simulink model "gm_MATE_HDLsolver_myFirstCircuit"  (R2024b)
settings: Solver=FixedStepDiscrete  StartTime=0.0  StopTime=0.05  FixedStep=6.02409638554217e-09  MaxStep=100e-6  RelTol=1e-4
PostLoadFcn:
  | Ts=1e-6; nb_sw=3; nb_lc=2;nb_r=1;nb_src=1; nb_out=3; rL=1.2;rC=100;L=1e-3; C=1e-5; LpejoSw=1e-6;h=Ts; MAX_INPUTS=16;
  | MAX_OUTPUTS=16;
  | MAX_SWITCHES=8;
  | MAX_INPUTS=16;
InitFcn:
  | Ts=1e-6; nb_sw=3; nb_lc=2;nb_r=1;nb_src=1; nb_out=3; rL=1.2;rC=100;L=1e-3; C=1e-5; LpejoSw=1e-6;h=Ts; MAX_INPUTS=16;
  | MAX_OUTPUTS=16;
  | MAX_SWITCHES=8;
  | MAX_INPUTS=16;
undefined symbols (not defined in the file or in its folder): MATE_SOC
libraries: fl_lib x31, nesl_utility x13, hdlmdlgenlib x10, simetranss x5, simulink x4, hdlsllib x3, ee_lib x2, eeGeneralControl x1
(part 3 of 8)

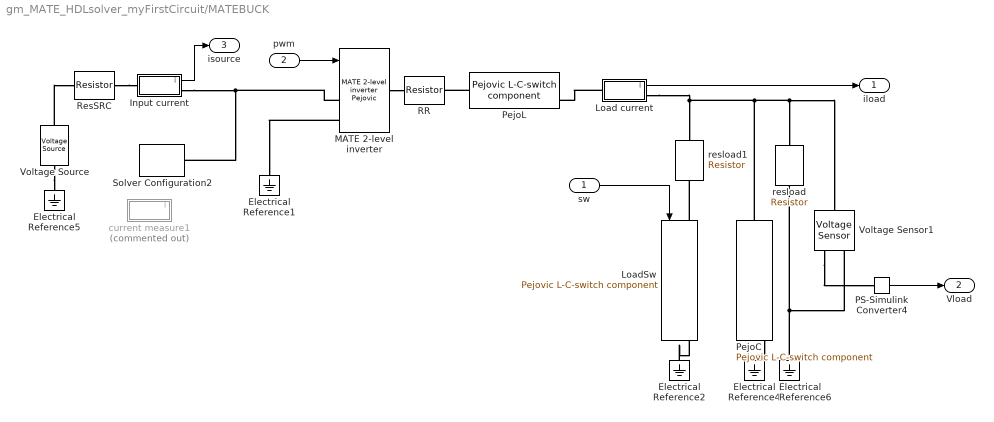
== system gm_MATE_HDLsolver_myFirstCircuit/MATEBUCK ==
  sw : Inport
  pwm : Inport  Port=2
  Electrical Reference{1..2,4..6} (5 alike) : fl_lib/Electrical/Electrical Elements/Electrical Reference
  Input current : Subsystem
  Load current : Subsystem
  LoadSw : simetranss/FPGA/Pejovic L-C-switch component  typ=Switch  Lon=LpejoSw  L=L  C=C  otherSW='coming soon'  Ts=Ts  pcbp=off
  MATE 2-level inverter : simetranss/FPGA/MATE 2-level inverter Pejovic  Lon=1e-6  Ts=Ts
  PS-Simulink Converter4 : nesl_utility/PS-Simulink Converter  PhysicalDomain=network_engine_domain  SubClassName=ps_output  LeftPortType=input  RightPortType=output  PseudoPeriodic=off  Frequencies=[]  VectorFormat=inherit  Unit=inherit  AffineConversion=off
  PejoC : simetranss/FPGA/Pejovic L-C-switch component  typ=Capacitor  Lon=LpejoSw  L=L  C=C  otherSW='coming soon'  Ts=Ts  pcbp=off
  PejoL : simetranss/FPGA/Pejovic L-C-switch component  typ=Inductor  Lon=LpejoSw  L=L  C=C  otherSW='coming soon'  Ts=Ts  pcbp=off
  RR : fl_lib/Electrical/Electrical Elements/Resistor  R=rL Ohm  i_specify=off  i_priority=None  i=0 A  i_nominal_specify=off  i_nominal_value=1  i_nominal_unit=A  v_specify=off  v_priority=None  v=0 V  v_nominal_specify=off  v_nominal_value=1  v_nominal_unit=V
  ResSRC : fl_lib/Electrical/Electrical Elements/Resistor  R=0.01 Ohm  i_specify=off  i_priority=None  i=0 A  i_nominal_specify=off  i_nominal_value=1  i_nominal_unit=A  v_specify=off  v_priority=None  v=0 V  v_nominal_specify=off  v_nominal_value=1  v_nominal_unit=V
  Solver Configuration2 : nesl_utility/Solver Configuration  PhysicalDomain=network_engine_domain  SubClassName=solver  LeftPortType=input  RightPortType=generic  Tones=[]  Harmonics=[]  SimulateNoise=off  Profile=off  UseLocalSampling=off  EnableSwitchedLinearOptims=on  FrequencyDomain=off  UseCCode=off  RelTol=0.001  AbsTol=0.001  MinStep=1e-09  ToWorkspace=off  RevertToSquareIcSolve=off  NumHomotopyIterations=100  PhasorMode=off  PhasorModeNumHarmonics=1  ConsistencySolver=NEWTON_XTOL_AFTER_FTOL  IndexReductionMethod=DerivativeReplacement  DoDC=off  ResidualTolerance=1e-09  ConsistencyTolSource=GLOBAL  ConsistencyAbsTol=0.001  ConsistencyRelTol=0.001  ConsistencyTolFactor=0.001  UseLocalSolver=on  LocalSolverChoice=NE_BACKWARD_EULER_ADVANCER  ResolveIndetEquations=on  FunctionEvalNumThread=1  LocalSolverSampleTime=Ts  DoFixedCost=on  MaxNonlinIter=1  MaxModeIter=2  ComputeImpulses=off  ImpulseIterations=2  LinearAlgebra=auto  LinearAlgebraNumThread=0  EquationFormulation=NE_TIME_EF  DelaysMemoryBudget=1024  AutomaticFiltering=on  FilteringTimeConstant=0.001  PartitionStorageMethod=AS_NEEDED  PartitionMemoryBudget=1024  PartitionMethod=ROBUST  MultibodyUseLocalSolver=off  MultibodyLocalSolverChoice=ODE1  MultibodyLocalSolverSampleTime=0.001
  Voltage Sensor1 : fl_lib/Electrical/Electrical Sensors/Voltage Sensor
  Voltage Source : ee_lib/Sources/Voltage Source  dc_voltage=100 V  ac_voltage=0 V  ac_shift=0 rad  ac_frequency=60 Hz  noise_mode=ee.enum.sources.noise.Disabled  PSD=0 V^2/Hz  sample_time=1e-3 s  repeatability=ee.enum.sources.repeatability.NotRepeatable  user_seed=0  auto_seed=136721035  i_specify=off  i_priority=None  i=0 A  i_nominal_specify=off  i_nominal_value=1  i_nominal_unit=A  v_specify=off  v_priority=None  v=0 V  v_nominal_specify=off  v_nominal_value=1  v_nominal_unit=V
  current measure1 : Subsystem  Commented=on
      mask Display: disp('amp')
  resload : fl_lib/Electrical/Electrical Elements/Resistor  R=rC Ohm  i_specify=off  i_priority=None  i=0 A  i_nominal_specify=off  i_nominal_value=1  i_nominal_unit=A  v_specify=off  v_priority=None  v=0 V  v_nominal_specify=off  v_nominal_value=1  v_nominal_unit=V
  resload1 : fl_lib/Electrical/Electrical Elements/Resistor  R=rC Ohm  i_specify=off  i_priority=None  i=0 A  i_nominal_specify=off  i_nominal_value=1  i_nominal_unit=A  v_specify=off  v_priority=None  v=0 V  v_nominal_specify=off  v_nominal_value=1  v_nominal_unit=V
  iload : Outport
  Vload : Outport  Port=2
  isource : Outport  Port=3
  wires:
  Input current/1(i) -> isource/1
  pwm/1 -> MATE 2-level inverter/1
  Load current/1(i) -> iload/1
  sw/1 -> LoadSw/1
  PS-Simulink Converter4/1 -> Vload/1
  connections:
  ResSRC/RConn1 -- Input current/LConn1
  Electrical Reference2/LConn1 -- LoadSw/RConn1
  LoadSw/LConn1 -- resload1/RConn1
  MATE 2-level inverter/LConn2 -- Electrical Reference1/LConn1
  PejoC/LConn1 -- resload1/LConn1 -- Load current/RConn1 -- resload/LConn1 -- Voltage Sensor1/LConn1
  Solver Configuration2/RConn1 -- MATE 2-level inverter/LConn1 -- Input current/RConn1
  Voltage Sensor1/RConn2 -- resload/RConn1 -- Electrical Reference6/LConn1
  Voltage Sensor1/RConn1 -- PS-Simulink Converter4/LConn1
  PejoC/RConn1 -- Electrical Reference4/LConn1
  PejoL/LConn1 -- RR/RConn1
  MATE 2-level inverter/RConn1 -- RR/LConn1
  Voltage Source/LConn1 -- ResSRC/LConn1
  Voltage Source/RConn1 -- Electrical Reference5/LConn1
  Load current/LConn1 -- PejoL/RConn1

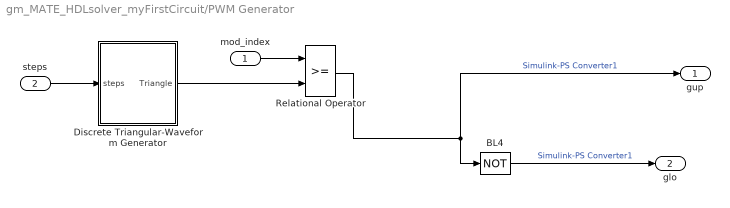
== system gm_MATE_HDLsolver_myFirstCircuit/PWM Generator ==
  mod_index : Inport
  steps : Inport  Port=2
  BL4 : Logic  Operator=NOT  Inputs=1
  Discrete Triangular-Waveform Generator : Subsystem
  Relational Operator : RelationalOperator  OutDataTypeStr=boolean
  gup : Outport  VectorParamsAs1DForOutWhenUnconnected=off
  glo : Outport  Port=2  VectorParamsAs1DForOutWhenUnconnected=off
  wires:
  BL4/1 -> glo/1  "Simulink-PS Converter1"
  Relational Operator/1 -> BL4/1, gup/1  "Simulink-PS Converter1"
  steps/1 -> Discrete Triangular-Waveform Generator/1(steps)
  mod_index/1 -> Relational Operator/1
  Discrete Triangular-Waveform Generator/1(Triangle) -> Relational Operator/2

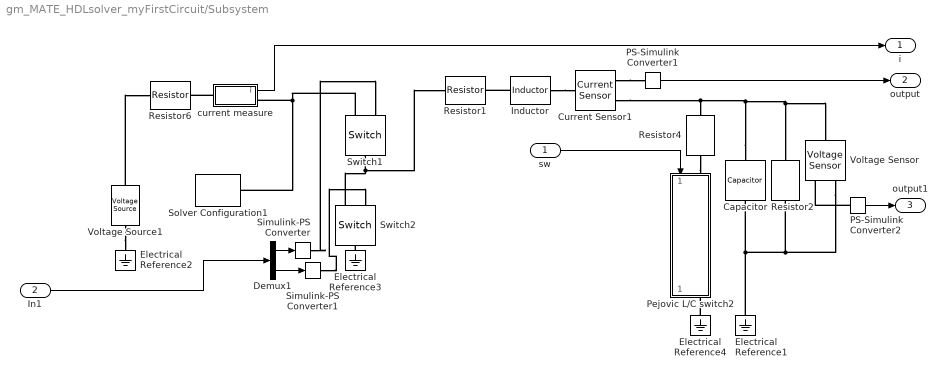
== system gm_MATE_HDLsolver_myFirstCircuit/Subsystem ==
  sw : Inport
  In1 : Inport  Port=2
  Capacitor : fl_lib/Electrical/Electrical Elements/Capacitor  c=C F  r=0 Ohm  g=0 1/Ohm  i_specify=off  i_priority=None  i=0 A  i_nominal_specify=off  i_nominal_value=1  i_nominal_unit=A  v_specify=off  v_priority=None  v=0 V  v_nominal_specify=off  v_nominal_value=1  v_nominal_unit=V  vc_specify=off  vc_priority=High  vc=0 V  vc_nominal_specify=off  vc_nominal_value=1  vc_nominal_unit=V
  Current Sensor1 : fl_lib/Electrical/Electrical Sensors/Current Sensor
  Demux1 : Demux  Outputs=2
  Electrical Reference{1..4} (4 alike) : fl_lib/Electrical/Electrical Elements/Electrical Reference
  Inductor : fl_lib/Electrical/Electrical Elements/Inductor  l=L H  r=0 Ohm  g=1e-9 1/Ohm  i_specify=off  i_priority=None  i=0 A  i_nominal_specify=off  i_nominal_value=1  i_nominal_unit=A  v_specify=off  v_priority=None  v=0 V  v_nominal_specify=off  v_nominal_value=1  v_nominal_unit=V  i_L_specify=off  i_L_priority=High  i_L=0 A  i_L_nominal_specify=off  i_L_nominal_value=1  i_L_nominal_unit=A
  PS-Simulink Converter1 : nesl_utility/PS-Simulink Converter  PhysicalDomain=network_engine_domain  SubClassName=ps_output  LeftPortType=input  RightPortType=output  PseudoPeriodic=off  Frequencies=[]  VectorFormat=inherit  Unit=inherit  AffineConversion=off
  PS-Simulink Converter2 : nesl_utility/PS-Simulink Converter  PhysicalDomain=network_engine_domain  SubClassName=ps_output  LeftPortType=input  RightPortType=output  PseudoPeriodic=off  Frequencies=[]  VectorFormat=inherit  Unit=inherit  AffineConversion=off
  Pejovic L/C switch2 : Subsystem  AncestorBlock=simetranss/FPGA/Pejovic L//C switch  mask(Pejovic Switch){Lon=LpejoSw, Ts=Ts}
      mask prompts: Lon "Selected equivalent ON inductance (H)"; Ts "Sample Time (s)"
      mask help:
      | Pejovic switch model in SimScape
      |
      | Implements a single phase switch model using the Pejovic constant admittance method.
      | The user only has to select the equivalent ON-state inductance of the model, the corresponding Capacitance is computed internally.
      |
      | In the Pejovic model, Ts/Lon=Coff/Ts (Backward Euler) resulting in a constant admittance for the DAE solver.
      |
      | Input signals;
      |
      | gate: the switch gate value (1 for ON , 0 for OFF)
      mask init:
      | Coff=Ts*Ts/Lon;
      | Rsw=Lon/Ts;
      | 
      | if Ts>2e-6
      |     warndlg(['Sample Time of ' num2str(Ts) ' s. may be somehow large for the Pejovic switch to be accurate. Sample time below 2 us are recommended.'])
      | end
      mask Display: disp(['Pswitch'])
  Resistor1 : fl_lib/Electrical/Electrical Elements/Resistor  R=rL Ohm  i_specify=off  i_priority=None  i=0 A  i_nominal_specify=off  i_nominal_value=1  i_nominal_unit=A  v_specify=off  v_priority=None  v=0 V  v_nominal_specify=off  v_nominal_value=1  v_nominal_unit=V
  Resistor2 : fl_lib/Electrical/Electrical Elements/Resistor  R=rC Ohm  i_specify=off  i_priority=None  i=0 A  i_nominal_specify=off  i_nominal_value=1  i_nominal_unit=A  v_specify=off  v_priority=None  v=0 V  v_nominal_specify=off  v_nominal_value=1  v_nominal_unit=V
  Resistor4 : fl_lib/Electrical/Electrical Elements/Resistor  R=rC Ohm  i_specify=off  i_priority=None  i=0 A  i_nominal_specify=off  i_nominal_value=1  i_nominal_unit=A  v_specify=off  v_priority=None  v=0 V  v_nominal_specify=off  v_nominal_value=1  v_nominal_unit=V
  Resistor6 : fl_lib/Electrical/Electrical Elements/Resistor  R=0.01 Ohm  i_specify=off  i_priority=None  i=0 A  i_nominal_specify=off  i_nominal_value=1  i_nominal_unit=A  v_specify=off  v_priority=None  v=0 V  v_nominal_specify=off  v_nominal_value=1  v_nominal_unit=V
  Simulink-PS Converter : nesl_utility/Simulink-PS Converter  PhysicalDomain=network_engine_domain  SubClassName=ps_input  LeftPortType=input  RightPortType=output  PseudoPeriodic=off  Frequencies=[]  NoiseDistribution=none  NoiseParameters=[]  Unit=1  AffineConversion=off  FilteringAndDerivatives=provide  SimscapeFilterOrder=1  InputFilterTimeConstant=0.001  UdotUserProvided=0
  Simulink-PS Converter1 : nesl_utility/Simulink-PS Converter  PhysicalDomain=network_engine_domain  SubClassName=ps_input  LeftPortType=input  RightPortType=output  PseudoPeriodic=off  Frequencies=[]  NoiseDistribution=none  NoiseParameters=[]  Unit=1  AffineConversion=off  FilteringAndDerivatives=provide  SimscapeFilterOrder=1  InputFilterTimeConstant=0.001  UdotUserProvided=0
  Solver Configuration1 : nesl_utility/Solver Configuration  PhysicalDomain=network_engine_domain  SubClassName=solver  LeftPortType=input  RightPortType=generic  Tones=[]  Harmonics=[]  SimulateNoise=off  Profile=off  UseLocalSampling=off  EnableSwitchedLinearOptims=on  FrequencyDomain=off  UseCCode=off  RelTol=0.001  AbsTol=0.001  MinStep=1e-09  ToWorkspace=off  RevertToSquareIcSolve=off  NumHomotopyIterations=100  PhasorMode=off  PhasorModeNumHarmonics=1  ConsistencySolver=NEWTON_XTOL_AFTER_FTOL  IndexReductionMethod=DerivativeReplacement  DoDC=off  ResidualTolerance=1e-09  ConsistencyTolSource=GLOBAL  ConsistencyAbsTol=0.001  ConsistencyRelTol=0.001  ConsistencyTolFactor=0.001  UseLocalSolver=on  LocalSolverChoice=NE_BACKWARD_EULER_ADVANCER  ResolveIndetEquations=on  FunctionEvalNumThread=1  LocalSolverSampleTime=Ts  DoFixedCost=on  MaxNonlinIter=1  MaxModeIter=2  ComputeImpulses=off  ImpulseIterations=2  LinearAlgebra=auto  LinearAlgebraNumThread=0  EquationFormulation=NE_TIME_EF  DelaysMemoryBudget=1024  AutomaticFiltering=on  FilteringTimeConstant=0.001  PartitionStorageMethod=AS_NEEDED  PartitionMemoryBudget=1024  PartitionMethod=ROBUST  MultibodyUseLocalSolver=off  MultibodyLocalSolverChoice=ODE1  MultibodyLocalSolverSampleTime=0.001
  Switch1 : fl_lib/Electrical/Electrical Elements/Switch  R_closed=0.001 Ohm  G_open=1e-8 1/Ohm  Threshold=0.5  i_specify=off  i_priority=None  i=0 A  i_nominal_specify=off  i_nominal_value=1  i_nominal_unit=A  v_specify=off  v_priority=None  v=0 V  v_nominal_specify=off  v_nominal_value=1  v_nominal_unit=V
  Switch2 : fl_lib/Electrical/Electrical Elements/Switch  R_closed=0.001 Ohm  G_open=1e-8 1/Ohm  Threshold=0.5  i_specify=off  i_priority=None  i=0 A  i_nominal_specify=off  i_nominal_value=1  i_nominal_unit=A  v_specify=off  v_priority=None  v=0 V  v_nominal_specify=off  v_nominal_value=1  v_nominal_unit=V
  Voltage Sensor : fl_lib/Electrical/Electrical Sensors/Voltage Sensor
  Voltage Source1 : ee_lib/Sources/Voltage Source  dc_voltage=100 V  ac_voltage=0 V  ac_shift=0 rad  ac_frequency=60 Hz  noise_mode=ee.enum.sources.noise.Disabled  PSD=0 V^2/Hz  sample_time=1e-3 s  repeatability=ee.enum.sources.repeatability.NotRepeatable  user_seed=0  auto_seed=1189375164  i_specify=off  i_priority=None  i=0 A  i_nominal_specify=off  i_nominal_value=1  i_nominal_unit=A  v_specify=off  v_priority=None  v=0 V  v_nominal_specify=off  v_nominal_value=1  v_nominal_unit=V
  current measure : Subsystem
      mask Display: disp('amp')
  i : Outport
  output : Outport  Port=2
  output1 : Outport  Port=3
  wires:
  PS-Simulink Converter2/1 -> output1/1
  PS-Simulink Converter1/1 -> output/1
  In1/1 -> Demux1/1
  Demux1/1 -> Simulink-PS Converter/1
  current measure/1(i) -> i/1
  Demux1/2 -> Simulink-PS Converter1/1
  sw/1 -> Pejovic L/C switch2/1(gate)
  connections:
  Voltage Source1/RConn1 -- Electrical Reference2/LConn1
  Electrical Reference3/LConn1 -- Switch2/LConn1
  Current Sensor1/RConn1 -- PS-Simulink Converter1/LConn1
  Inductor/LConn1 -- Resistor1/RConn1
  Inductor/RConn1 -- Current Sensor1/LConn1
  Simulink-PS Converter1/RConn1 -- Switch2/RConn1
  PS-Simulink Converter2/LConn1 -- Voltage Sensor/RConn1
  Voltage Source1/LConn1 -- Resistor6/LConn1
  current measure/LConn1 -- Resistor6/RConn1
  Resistor4/RConn1 -- Pejovic L/C switch2/LConn1
  Electrical Reference1/LConn1 -- Capacitor/RConn1 -- Resistor2/RConn1 -- Voltage Sensor/RConn2
  Capacitor/LConn1 -- Resistor2/LConn1 -- Voltage Sensor/LConn1 -- Resistor4/LConn1 -- Current Sensor1/RConn2
  Switch1/LConn1 -- Resistor1/LConn1 -- Switch2/RConn2
  Solver Configuration1/RConn1 -- current measure/RConn1 -- Switch1/RConn2
  Simulink-PS Converter/RConn1 -- Switch1/RConn1
  Electrical Reference4/LConn1 -- Pejovic L/C switch2/RConn1

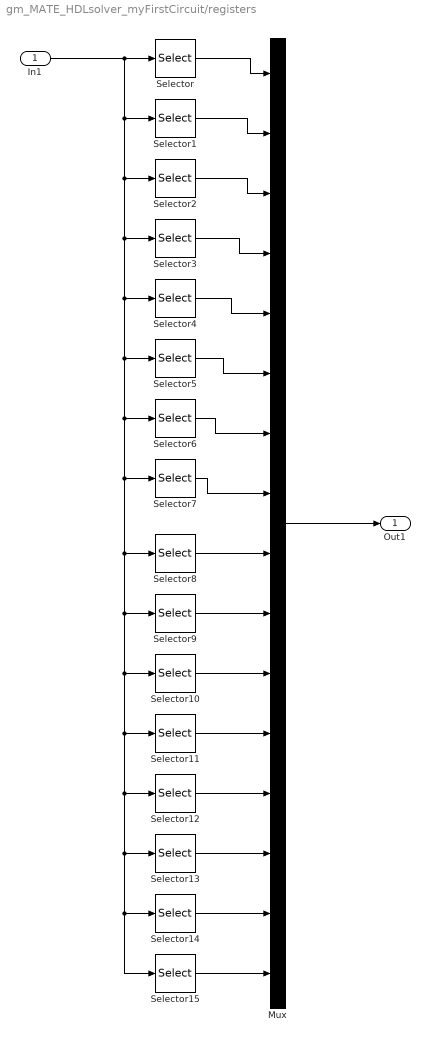
== system gm_MATE_HDLsolver_myFirstCircuit/registers ==
  In1 : Inport
  Mux : Mux  Inputs=16
  Selector : Selector  InputPortWidth=16  IndexOptions=Index vector (dialog)  Indices=1  OutputSizes=1
  Selector1 : Selector  InputPortWidth=16  IndexOptions=Index vector (dialog)  Indices=2  OutputSizes=1
  Selector10 : Selector  InputPortWidth=16  IndexOptions=Index vector (dialog)  Indices=11  OutputSizes=1
  Selector11 : Selector  InputPortWidth=16  IndexOptions=Index vector (dialog)  Indices=12  OutputSizes=1
  Selector12 : Selector  InputPortWidth=16  IndexOptions=Index vector (dialog)  Indices=13  OutputSizes=1
  Selector13 : Selector  InputPortWidth=16  IndexOptions=Index vector (dialog)  Indices=14  OutputSizes=1
  Selector14 : Selector  InputPortWidth=16  IndexOptions=Index vector (dialog)  Indices=15  OutputSizes=1
  Selector15 : Selector  InputPortWidth=16  IndexOptions=Index vector (dialog)  Indices=16  OutputSizes=1
  Selector2 : Selector  InputPortWidth=16  IndexOptions=Index vector (dialog)  Indices=3  OutputSizes=1
  Selector3 : Selector  InputPortWidth=16  IndexOptions=Index vector (dialog)  Indices=4  OutputSizes=1
  Selector4 : Selector  InputPortWidth=16  IndexOptions=Index vector (dialog)  Indices=5  OutputSizes=1
  Selector5 : Selector  InputPortWidth=16  IndexOptions=Index vector (dialog)  Indices=6  OutputSizes=1
  Selector6 : Selector  InputPortWidth=16  IndexOptions=Index vector (dialog)  Indices=7  OutputSizes=1
  Selector7 : Selector  InputPortWidth=16  IndexOptions=Index vector (dialog)  Indices=8  OutputSizes=1
  Selector8 : Selector  InputPortWidth=16  IndexOptions=Index vector (dialog)  Indices=9  OutputSizes=1
  Selector9 : Selector  InputPortWidth=16  IndexOptions=Index vector (dialog)  Indices=10  OutputSizes=1
  Out1 : Outport
  wires:
  Mux/1 -> Out1/1
  Selector7/1 -> Mux/8
  Selector6/1 -> Mux/7
  Selector5/1 -> Mux/6
  Selector4/1 -> Mux/5
  Selector3/1 -> Mux/4
  Selector2/1 -> Mux/3
  Selector1/1 -> Mux/2
  Selector/1 -> Mux/1
  Selector15/1 -> Mux/16
  Selector14/1 -> Mux/15
  Selector13/1 -> Mux/14
  Selector12/1 -> Mux/13
  Selector11/1 -> Mux/12
  Selector10/1 -> Mux/11
  Selector9/1 -> Mux/10
  Selector8/1 -> Mux/9
  In1/1 -> Selector14/1, Selector15/1, Selector13/1, Selector12/1, Selector11/1, Selector10/1, Selector9/1, Selector8/1, Selector7/1, Selector6/1, Selector5/1, Selector4/1, Selector3/1, Selector2/1, Selector1/1, Selector/1

== system gm_MATE_HDLsolver_myFirstCircuit/ForFPGA/Compare To Constant ==
  u : Inport  OutDataTypeStr=fixdt(0,8,0,'DataTypeOverride', 'Off')  SampleTime=1e-06
  Compare : RelationalOperator  Operator===  OutDataTypeStr=boolean
  Constant : Constant  DisableCoverage=on  Value=const  OutDataTypeStr=uint8  SampleTime=-1
  y : Outport  SampleTime=1e-06
  wires:
  u/1 -> Compare/1
  Compare/1 -> y/1
  Constant/1 -> Compare/2

== system gm_MATE_HDLsolver_myFirstCircuit/ForFPGA/Counter Free-Running ==
  Force to be scalar : SignalSpecification  OutDataTypeStr=fixdt(0, 4, 0)  Dimensions=1
  Increment Real World : Subsystem  mask(Real World Value Increment){}
      mask help: Simulink:masks:RealWorldValueIncrement_MD
      mask Display: disp('V++')
  Output : Delay  DelayLength=double(1)  InitialCondition=0  SampleTime=1e-06
  Wrap To Zero : Subsystem  mask(Wrap To Zero){Threshold=double(15)}
      mask prompts: Threshold "Simulink:masks:Threshold_MP"
      mask help: Simulink:masks:WrapToZero_MD
  y : Outport  SampleTime=1e-06
  wires:
  Wrap To Zero/1(Y) -> Output/1
  Output/1 -> y/1, Force to be scalar/1
  Increment Real World/1(y) -> Wrap To Zero/1(U)
  Force to be scalar/1 -> Increment Real World/1(u)

== system gm_MATE_HDLsolver_myFirstCircuit/ForFPGA/Dot Product ==
  In1 : Inport
  In2 : Inport  Port=2
  Dot Product : Sum  OutDataTypeStr=single  SampleTime=6.02409638554217e-09
  Dot Product_pd1 : Delay  DelayLength=6
  Out1 : Outport
  wires:
  In1/1 -> Dot Product/1
  In2/1 -> Dot Product/2
  Dot Product/1 -> Dot Product_pd1/1
  Dot Product_pd1/1 -> Out1/1

== system gm_MATE_HDLsolver_myFirstCircuit/ForFPGA/Dot Product1 ==
  In1 : Inport
  In2 : Inport  Port=2
  Dot Product1 : Sum  OutDataTypeStr=single  SampleTime=6.02409638554217e-09
  Dot Product1_pd1 : Delay  DelayLength=6
  Out1 : Outport
  wires:
  In1/1 -> Dot Product1/1
  In2/1 -> Dot Product1/2
  Dot Product1/1 -> Dot Product1_pd1/1
  Dot Product1_pd1/1 -> Out1/1

== system gm_MATE_HDLsolver_myFirstCircuit/ForFPGA/Dot Product10 ==
  In1 : Inport
  In2 : Inport  Port=2
  Dot Product10 : Sum  OutDataTypeStr=single  SampleTime=6.02409638554217e-09
  Dot Product10_pd1 : Delay  DelayLength=6
  Out1 : Outport
  wires:
  In1/1 -> Dot Product10/1
  In2/1 -> Dot Product10/2
  Dot Product10/1 -> Dot Product10_pd1/1
  Dot Product10_pd1/1 -> Out1/1

== system gm_MATE_HDLsolver_myFirstCircuit/ForFPGA/Dot Product101 ==
  In1 : Inport
  In2 : Inport  Port=2
  Dot Product101 : Sum  OutDataTypeStr=single  SampleTime=6.02409638554217e-09
  Dot Product101_pd1 : Delay  DelayLength=6
  Out1 : Outport
  wires:
  In1/1 -> Dot Product101/1
  In2/1 -> Dot Product101/2
  Dot Product101/1 -> Dot Product101_pd1/1
  Dot Product101_pd1/1 -> Out1/1

== system gm_MATE_HDLsolver_myFirstCircuit/ForFPGA/Dot Product1010 ==
  In1 : Inport
  In2 : Inport  Port=2
  Dot Product1010 : Sum  OutDataTypeStr=single  SampleTime=6.02409638554217e-09
  Dot Product1010_pd1 : Delay  DelayLength=6
  Out1 : Outport
  wires:
  In1/1 -> Dot Product1010/1
  In2/1 -> Dot Product1010/2
  Dot Product1010/1 -> Dot Product1010_pd1/1
  Dot Product1010_pd1/1 -> Out1/1

== system gm_MATE_HDLsolver_myFirstCircuit/ForFPGA/Dot Product1011 ==
  In1 : Inport
  In2 : Inport  Port=2
  Dot Product1011 : Sum  OutDataTypeStr=single  SampleTime=6.02409638554217e-09
  Dot Product1011_pd1 : Delay  DelayLength=6
  Out1 : Outport
  wires:
  In1/1 -> Dot Product1011/1
  In2/1 -> Dot Product1011/2
  Dot Product1011/1 -> Dot Product1011_pd1/1
  Dot Product1011_pd1/1 -> Out1/1

== system gm_MATE_HDLsolver_myFirstCircuit/ForFPGA/Dot Product1012 ==
  In1 : Inport
  In2 : Inport  Port=2
  Dot Product1012 : Sum  OutDataTypeStr=single  SampleTime=6.02409638554217e-09
  Dot Product1012_pd1 : Delay  DelayLength=6
  Out1 : Outport
  wires:
  In1/1 -> Dot Product1012/1
  In2/1 -> Dot Product1012/2
  Dot Product1012/1 -> Dot Product1012_pd1/1
  Dot Product1012_pd1/1 -> Out1/1

== system gm_MATE_HDLsolver_myFirstCircuit/ForFPGA/Dot Product1013 ==
  In1 : Inport
  In2 : Inport  Port=2
  Dot Product1013 : Sum  OutDataTypeStr=single  SampleTime=6.02409638554217e-09
  Dot Product1013_pd1 : Delay  DelayLength=6
  Out1 : Outport
  wires:
  In1/1 -> Dot Product1013/1
  In2/1 -> Dot Product1013/2
  Dot Product1013/1 -> Dot Product1013_pd1/1
  Dot Product1013_pd1/1 -> Out1/1

== system gm_MATE_HDLsolver_myFirstCircuit/ForFPGA/Dot Product1014 ==
  In1 : Inport
  In2 : Inport  Port=2
  Dot Product1014 : Sum  OutDataTypeStr=single  SampleTime=6.02409638554217e-09
  Dot Product1014_pd1 : Delay  DelayLength=6
  Out1 : Outport
  wires:
  In1/1 -> Dot Product1014/1
  In2/1 -> Dot Product1014/2
  Dot Product1014/1 -> Dot Product1014_pd1/1
  Dot Product1014_pd1/1 -> Out1/1

== system gm_MATE_HDLsolver_myFirstCircuit/ForFPGA/Dot Product1015 ==
  In1 : Inport
  In2 : Inport  Port=2
  Dot Product1015 : Sum  OutDataTypeStr=single  SampleTime=6.02409638554217e-09
  Dot Product1015_pd1 : Delay  DelayLength=6
  Out1 : Outport
  wires:
  In1/1 -> Dot Product1015/1
  In2/1 -> Dot Product1015/2
  Dot Product1015/1 -> Dot Product1015_pd1/1
  Dot Product1015_pd1/1 -> Out1/1

== system gm_MATE_HDLsolver_myFirstCircuit/ForFPGA/Dot Product102 ==
  In1 : Inport
  In2 : Inport  Port=2
  Dot Product102 : Sum  OutDataTypeStr=single  SampleTime=6.02409638554217e-09
  Dot Product102_pd1 : Delay  DelayLength=6
  Out1 : Outport
  wires:
  In1/1 -> Dot Product102/1
  In2/1 -> Dot Product102/2
  Dot Product102/1 -> Dot Product102_pd1/1
  Dot Product102_pd1/1 -> Out1/1

== system gm_MATE_HDLsolver_myFirstCircuit/ForFPGA/Dot Product103 ==
  In1 : Inport
  In2 : Inport  Port=2
  Dot Product103 : Sum  OutDataTypeStr=single  SampleTime=6.02409638554217e-09
  Dot Product103_pd1 : Delay  DelayLength=6
  Out1 : Outport
  wires:
  In1/1 -> Dot Product103/1
  In2/1 -> Dot Product103/2
  Dot Product103/1 -> Dot Product103_pd1/1
  Dot Product103_pd1/1 -> Out1/1

== system gm_MATE_HDLsolver_myFirstCircuit/ForFPGA/Dot Product104 ==
  In1 : Inport
  In2 : Inport  Port=2
  Dot Product104 : Sum  OutDataTypeStr=single  SampleTime=6.02409638554217e-09
  Dot Product104_pd1 : Delay  DelayLength=6
  Out1 : Outport
  wires:
  In1/1 -> Dot Product104/1
  In2/1 -> Dot Product104/2
  Dot Product104/1 -> Dot Product104_pd1/1
  Dot Product104_pd1/1 -> Out1/1

== system gm_MATE_HDLsolver_myFirstCircuit/ForFPGA/Dot Product105 ==
  In1 : Inport
  In2 : Inport  Port=2
  Dot Product105 : Sum  OutDataTypeStr=single  SampleTime=6.02409638554217e-09
  Dot Product105_pd1 : Delay  DelayLength=6
  Out1 : Outport
  wires:
  In1/1 -> Dot Product105/1
  In2/1 -> Dot Product105/2
  Dot Product105/1 -> Dot Product105_pd1/1
  Dot Product105_pd1/1 -> Out1/1

== system gm_MATE_HDLsolver_myFirstCircuit/ForFPGA/Dot Product106 ==
  In1 : Inport
  In2 : Inport  Port=2
  Dot Product106 : Sum  OutDataTypeStr=single  SampleTime=6.02409638554217e-09
  Dot Product106_pd1 : Delay  DelayLength=6
  Out1 : Outport
  wires:
  In1/1 -> Dot Product106/1
  In2/1 -> Dot Product106/2
  Dot Product106/1 -> Dot Product106_pd1/1
  Dot Product106_pd1/1 -> Out1/1

== system gm_MATE_HDLsolver_myFirstCircuit/ForFPGA/Dot Product107 ==
  In1 : Inport
  In2 : Inport  Port=2
  Dot Product107 : Sum  OutDataTypeStr=single  SampleTime=6.02409638554217e-09
  Dot Product107_pd1 : Delay  DelayLength=6
  Out1 : Outport
  wires:
  In1/1 -> Dot Product107/1
  In2/1 -> Dot Product107/2
  Dot Product107/1 -> Dot Product107_pd1/1
  Dot Product107_pd1/1 -> Out1/1

== system gm_MATE_HDLsolver_myFirstCircuit/ForFPGA/Dot Product108 ==
  In1 : Inport
  In2 : Inport  Port=2
  Dot Product108 : Sum  OutDataTypeStr=single  SampleTime=6.02409638554217e-09
  Dot Product108_pd1 : Delay  DelayLength=6
  Out1 : Outport
  wires:
  In1/1 -> Dot Product108/1
  In2/1 -> Dot Product108/2
  Dot Product108/1 -> Dot Product108_pd1/1
  Dot Product108_pd1/1 -> Out1/1

== system gm_MATE_HDLsolver_myFirstCircuit/ForFPGA/Dot Product109 ==
  In1 : Inport
  In2 : Inport  Port=2
  Dot Product109 : Sum  OutDataTypeStr=single  SampleTime=6.02409638554217e-09
  Dot Product109_pd1 : Delay  DelayLength=6
  Out1 : Outport
  wires:
  In1/1 -> Dot Product109/1
  In2/1 -> Dot Product109/2
  Dot Product109/1 -> Dot Product109_pd1/1
  Dot Product109_pd1/1 -> Out1/1

== system gm_MATE_HDLsolver_myFirstCircuit/ForFPGA/Dot Product11 ==
  In1 : Inport
  In2 : Inport  Port=2
  Dot Product11 : Sum  OutDataTypeStr=single  SampleTime=6.02409638554217e-09
  Dot Product11_pd1 : Delay  DelayLength=6
  Out1 : Outport
  wires:
  In1/1 -> Dot Product11/1
  In2/1 -> Dot Product11/2
  Dot Product11/1 -> Dot Product11_pd1/1
  Dot Product11_pd1/1 -> Out1/1

== system gm_MATE_HDLsolver_myFirstCircuit/ForFPGA/Dot Product110 ==
  In1 : Inport
  In2 : Inport  Port=2
  Dot Product110 : Sum  OutDataTypeStr=single  SampleTime=6.02409638554217e-09
  Dot Product110_pd1 : Delay  DelayLength=6
  Out1 : Outport
  wires:
  In1/1 -> Dot Product110/1
  In2/1 -> Dot Product110/2
  Dot Product110/1 -> Dot Product110_pd1/1
  Dot Product110_pd1/1 -> Out1/1

== system gm_MATE_HDLsolver_myFirstCircuit/ForFPGA/Dot Product111 ==
  In1 : Inport
  In2 : Inport  Port=2
  Dot Product111 : Sum  OutDataTypeStr=single  SampleTime=6.02409638554217e-09
  Dot Product111_pd1 : Delay  DelayLength=6
  Out1 : Outport
  wires:
  In1/1 -> Dot Product111/1
  In2/1 -> Dot Product111/2
  Dot Product111/1 -> Dot Product111_pd1/1
  Dot Product111_pd1/1 -> Out1/1

== system gm_MATE_HDLsolver_myFirstCircuit/ForFPGA/Dot Product1110 ==
  In1 : Inport
  In2 : Inport  Port=2
  Dot Product1110 : Sum  OutDataTypeStr=single  SampleTime=6.02409638554217e-09
  Dot Product1110_pd1 : Delay  DelayLength=6
  Out1 : Outport
  wires:
  In1/1 -> Dot Product1110/1
  In2/1 -> Dot Product1110/2
  Dot Product1110/1 -> Dot Product1110_pd1/1
  Dot Product1110_pd1/1 -> Out1/1

== system gm_MATE_HDLsolver_myFirstCircuit/ForFPGA/Dot Product1111 ==
  In1 : Inport
  In2 : Inport  Port=2
  Dot Product1111 : Sum  OutDataTypeStr=single  SampleTime=6.02409638554217e-09
  Dot Product1111_pd1 : Delay  DelayLength=6
  Out1 : Outport
  wires:
  In1/1 -> Dot Product1111/1
  In2/1 -> Dot Product1111/2
  Dot Product1111/1 -> Dot Product1111_pd1/1
  Dot Product1111_pd1/1 -> Out1/1

== system gm_MATE_HDLsolver_myFirstCircuit/ForFPGA/Dot Product1112 ==
  In1 : Inport
  In2 : Inport  Port=2
  Dot Product1112 : Sum  OutDataTypeStr=single  SampleTime=6.02409638554217e-09
  Dot Product1112_pd1 : Delay  DelayLength=6
  Out1 : Outport
  wires:
  In1/1 -> Dot Product1112/1
  In2/1 -> Dot Product1112/2
  Dot Product1112/1 -> Dot Product1112_pd1/1
  Dot Product1112_pd1/1 -> Out1/1

== system gm_MATE_HDLsolver_myFirstCircuit/ForFPGA/Dot Product1113 ==
  In1 : Inport
  In2 : Inport  Port=2
  Dot Product1113 : Sum  OutDataTypeStr=single  SampleTime=6.02409638554217e-09
  Dot Product1113_pd1 : Delay  DelayLength=6
  Out1 : Outport
  wires:
  In1/1 -> Dot Product1113/1
  In2/1 -> Dot Product1113/2
  Dot Product1113/1 -> Dot Product1113_pd1/1
  Dot Product1113_pd1/1 -> Out1/1

== system gm_MATE_HDLsolver_myFirstCircuit/ForFPGA/Dot Product1114 ==
  In1 : Inport
  In2 : Inport  Port=2
  Dot Product1114 : Sum  OutDataTypeStr=single  SampleTime=6.02409638554217e-09
  Dot Product1114_pd1 : Delay  DelayLength=6
  Out1 : Outport
  wires:
  In1/1 -> Dot Product1114/1
  In2/1 -> Dot Product1114/2
  Dot Product1114/1 -> Dot Product1114_pd1/1
  Dot Product1114_pd1/1 -> Out1/1

== system gm_MATE_HDLsolver_myFirstCircuit/ForFPGA/Dot Product1115 ==
  In1 : Inport
  In2 : Inport  Port=2
  Dot Product1115 : Sum  OutDataTypeStr=single  SampleTime=6.02409638554217e-09
  Dot Product1115_pd1 : Delay  DelayLength=6
  Out1 : Outport
  wires:
  In1/1 -> Dot Product1115/1
  In2/1 -> Dot Product1115/2
  Dot Product1115/1 -> Dot Product1115_pd1/1
  Dot Product1115_pd1/1 -> Out1/1

== system gm_MATE_HDLsolver_myFirstCircuit/ForFPGA/Dot Product1116 ==
  In1 : Inport
  In2 : Inport  Port=2
  Dot Product1116 : Sum  OutDataTypeStr=single  SampleTime=6.02409638554217e-09
  Dot Product1116_pd1 : Delay  DelayLength=6
  Out1 : Outport
  wires:
  In1/1 -> Dot Product1116/1
  In2/1 -> Dot Product1116/2
  Dot Product1116/1 -> Dot Product1116_pd1/1
  Dot Product1116_pd1/1 -> Out1/1

== system gm_MATE_HDLsolver_myFirstCircuit/ForFPGA/Dot Product1117 ==
  In1 : Inport
  In2 : Inport  Port=2
  Dot Product1117 : Sum  OutDataTypeStr=single  SampleTime=6.02409638554217e-09
  Dot Product1117_pd1 : Delay  DelayLength=6
  Out1 : Outport
  wires:
  In1/1 -> Dot Product1117/1
  In2/1 -> Dot Product1117/2
  Dot Product1117/1 -> Dot Product1117_pd1/1
  Dot Product1117_pd1/1 -> Out1/1

== system gm_MATE_HDLsolver_myFirstCircuit/ForFPGA/Dot Product1118 ==
  In1 : Inport
  In2 : Inport  Port=2
  Dot Product1118 : Sum  OutDataTypeStr=single  SampleTime=6.02409638554217e-09
  Dot Product1118_pd1 : Delay  DelayLength=6
  Out1 : Outport
  wires:
  In1/1 -> Dot Product1118/1
  In2/1 -> Dot Product1118/2
  Dot Product1118/1 -> Dot Product1118_pd1/1
  Dot Product1118_pd1/1 -> Out1/1

== system gm_MATE_HDLsolver_myFirstCircuit/ForFPGA/Dot Product1119 ==
  In1 : Inport
  In2 : Inport  Port=2
  Dot Product1119 : Sum  OutDataTypeStr=single  SampleTime=6.02409638554217e-09
  Dot Product1119_pd1 : Delay  DelayLength=6
  Out1 : Outport
  wires:
  In1/1 -> Dot Product1119/1
  In2/1 -> Dot Product1119/2
  Dot Product1119/1 -> Dot Product1119_pd1/1
  Dot Product1119_pd1/1 -> Out1/1

== system gm_MATE_HDLsolver_myFirstCircuit/ForFPGA/Dot Product112 ==
  In1 : Inport
  In2 : Inport  Port=2
  Dot Product112 : Sum  OutDataTypeStr=single  SampleTime=6.02409638554217e-09
  Dot Product112_pd1 : Delay  DelayLength=6
  Out1 : Outport
  wires:
  In1/1 -> Dot Product112/1
  In2/1 -> Dot Product112/2
  Dot Product112/1 -> Dot Product112_pd1/1
  Dot Product112_pd1/1 -> Out1/1

== system gm_MATE_HDLsolver_myFirstCircuit/ForFPGA/Dot Product1120 ==
  In1 : Inport
  In2 : Inport  Port=2
  Dot Product1120 : Sum  OutDataTypeStr=single  SampleTime=6.02409638554217e-09
  Dot Product1120_pd1 : Delay  DelayLength=6
  Out1 : Outport
  wires:
  In1/1 -> Dot Product1120/1
  In2/1 -> Dot Product1120/2
  Dot Product1120/1 -> Dot Product1120_pd1/1
  Dot Product1120_pd1/1 -> Out1/1

== system gm_MATE_HDLsolver_myFirstCircuit/ForFPGA/Dot Product1121 ==
  In1 : Inport
  In2 : Inport  Port=2
  Dot Product1121 : Sum  OutDataTypeStr=single  SampleTime=6.02409638554217e-09
  Dot Product1121_pd1 : Delay  DelayLength=6
  Out1 : Outport
  wires:
  In1/1 -> Dot Product1121/1
  In2/1 -> Dot Product1121/2
  Dot Product1121/1 -> Dot Product1121_pd1/1
  Dot Product1121_pd1/1 -> Out1/1

== system gm_MATE_HDLsolver_myFirstCircuit/ForFPGA/Dot Product1122 ==
  In1 : Inport
  In2 : Inport  Port=2
  Dot Product1122 : Sum  OutDataTypeStr=single  SampleTime=6.02409638554217e-09
  Dot Product1122_pd1 : Delay  DelayLength=6
  Out1 : Outport
  wires:
  In1/1 -> Dot Product1122/1
  In2/1 -> Dot Product1122/2
  Dot Product1122/1 -> Dot Product1122_pd1/1
  Dot Product1122_pd1/1 -> Out1/1

== system gm_MATE_HDLsolver_myFirstCircuit/ForFPGA/Dot Product1123 ==
  In1 : Inport
  In2 : Inport  Port=2
  Dot Product1123 : Sum  OutDataTypeStr=single  SampleTime=6.02409638554217e-09
  Dot Product1123_pd1 : Delay  DelayLength=6
  Out1 : Outport
  wires:
  In1/1 -> Dot Product1123/1
  In2/1 -> Dot Product1123/2
  Dot Product1123/1 -> Dot Product1123_pd1/1
  Dot Product1123_pd1/1 -> Out1/1

== system gm_MATE_HDLsolver_myFirstCircuit/ForFPGA/Dot Product1124 ==
  In1 : Inport
  In2 : Inport  Port=2
  Dot Product1124 : Sum  OutDataTypeStr=single  SampleTime=6.02409638554217e-09
  Dot Product1124_pd1 : Delay  DelayLength=6
  Out1 : Outport
  wires:
  In1/1 -> Dot Product1124/1
  In2/1 -> Dot Product1124/2
  Dot Product1124/1 -> Dot Product1124_pd1/1
  Dot Product1124_pd1/1 -> Out1/1

== system gm_MATE_HDLsolver_myFirstCircuit/ForFPGA/Dot Product113 ==
  In1 : Inport
  In2 : Inport  Port=2
  Dot Product113 : Sum  OutDataTypeStr=single  SampleTime=6.02409638554217e-09
  Dot Product113_pd1 : Delay  DelayLength=6
  Out1 : Outport
  wires:
  In1/1 -> Dot Product113/1
  In2/1 -> Dot Product113/2
  Dot Product113/1 -> Dot Product113_pd1/1
  Dot Product113_pd1/1 -> Out1/1

== system gm_MATE_HDLsolver_myFirstCircuit/ForFPGA/Dot Product114 ==
  In1 : Inport
  In2 : Inport  Port=2
  Dot Product114 : Sum  OutDataTypeStr=single  SampleTime=6.02409638554217e-09
  Dot Product114_pd1 : Delay  DelayLength=6
  Out1 : Outport
  wires:
  In1/1 -> Dot Product114/1
  In2/1 -> Dot Product114/2
  Dot Product114/1 -> Dot Product114_pd1/1
  Dot Product114_pd1/1 -> Out1/1

== system gm_MATE_HDLsolver_myFirstCircuit/ForFPGA/Dot Product115 ==
  In1 : Inport
  In2 : Inport  Port=2
  Dot Product115 : Sum  OutDataTypeStr=single  SampleTime=6.02409638554217e-09
  Dot Product115_pd1 : Delay  DelayLength=6
  Out1 : Outport
  wires:
  In1/1 -> Dot Product115/1
  In2/1 -> Dot Product115/2
  Dot Product115/1 -> Dot Product115_pd1/1
  Dot Product115_pd1/1 -> Out1/1

== system gm_MATE_HDLsolver_myFirstCircuit/ForFPGA/Dot Product116 ==
  In1 : Inport
  In2 : Inport  Port=2
  Dot Product116 : Sum  OutDataTypeStr=single  SampleTime=6.02409638554217e-09
  Dot Product116_pd1 : Delay  DelayLength=6
  Out1 : Outport
  wires:
  In1/1 -> Dot Product116/1
  In2/1 -> Dot Product116/2
  Dot Product116/1 -> Dot Product116_pd1/1
  Dot Product116_pd1/1 -> Out1/1

== system gm_MATE_HDLsolver_myFirstCircuit/ForFPGA/Dot Product117 ==
  In1 : Inport
  In2 : Inport  Port=2
  Dot Product117 : Sum  OutDataTypeStr=single  SampleTime=6.02409638554217e-09
  Dot Product117_pd1 : Delay  DelayLength=6
  Out1 : Outport
  wires:
  In1/1 -> Dot Product117/1
  In2/1 -> Dot Product117/2
  Dot Product117/1 -> Dot Product117_pd1/1
  Dot Product117_pd1/1 -> Out1/1

== system gm_MATE_HDLsolver_myFirstCircuit/ForFPGA/Dot Product118 ==
  In1 : Inport
  In2 : Inport  Port=2
  Dot Product118 : Sum  OutDataTypeStr=single  SampleTime=6.02409638554217e-09
  Dot Product118_pd1 : Delay  DelayLength=6
  Out1 : Outport
  wires:
  In1/1 -> Dot Product118/1
  In2/1 -> Dot Product118/2
  Dot Product118/1 -> Dot Product118_pd1/1
  Dot Product118_pd1/1 -> Out1/1

== system gm_MATE_HDLsolver_myFirstCircuit/ForFPGA/Dot Product119 ==
  In1 : Inport
  In2 : Inport  Port=2
  Dot Product119 : Sum  OutDataTypeStr=single  SampleTime=6.02409638554217e-09
  Dot Product119_pd1 : Delay  DelayLength=6
  Out1 : Outport
  wires:
  In1/1 -> Dot Product119/1
  In2/1 -> Dot Product119/2
  Dot Product119/1 -> Dot Product119_pd1/1
  Dot Product119_pd1/1 -> Out1/1

== system gm_MATE_HDLsolver_myFirstCircuit/ForFPGA/Dot Product12 ==
  In1 : Inport
  In2 : Inport  Port=2
  Dot Product12 : Sum  OutDataTypeStr=single  SampleTime=6.02409638554217e-09
  Dot Product12_pd1 : Delay  DelayLength=6
  Out1 : Outport
  wires:
  In1/1 -> Dot Product12/1
  In2/1 -> Dot Product12/2
  Dot Product12/1 -> Dot Product12_pd1/1
  Dot Product12_pd1/1 -> Out1/1

== system gm_MATE_HDLsolver_myFirstCircuit/ForFPGA/Dot Product121 ==
  In1 : Inport
  In2 : Inport  Port=2
  Dot Product121 : Sum  OutDataTypeStr=single  SampleTime=6.02409638554217e-09
  Dot Product121_pd1 : Delay  DelayLength=6
  Out1 : Outport
  wires:
  In1/1 -> Dot Product121/1
  In2/1 -> Dot Product121/2
  Dot Product121/1 -> Dot Product121_pd1/1
  Dot Product121_pd1/1 -> Out1/1

== system gm_MATE_HDLsolver_myFirstCircuit/ForFPGA/Dot Product1210 ==
  In1 : Inport
  In2 : Inport  Port=2
  Dot Product1210 : Sum  OutDataTypeStr=single  SampleTime=6.02409638554217e-09
  Dot Product1210_pd1 : Delay  DelayLength=6
  Out1 : Outport
  wires:
  In1/1 -> Dot Product1210/1
  In2/1 -> Dot Product1210/2
  Dot Product1210/1 -> Dot Product1210_pd1/1
  Dot Product1210_pd1/1 -> Out1/1

== system gm_MATE_HDLsolver_myFirstCircuit/ForFPGA/Dot Product1211 ==
  In1 : Inport
  In2 : Inport  Port=2
  Dot Product1211 : Sum  OutDataTypeStr=single  SampleTime=6.02409638554217e-09
  Dot Product1211_pd1 : Delay  DelayLength=6
  Out1 : Outport
  wires:
  In1/1 -> Dot Product1211/1
  In2/1 -> Dot Product1211/2
  Dot Product1211/1 -> Dot Product1211_pd1/1
  Dot Product1211_pd1/1 -> Out1/1

== system gm_MATE_HDLsolver_myFirstCircuit/ForFPGA/Dot Product1212 ==
  In1 : Inport
  In2 : Inport  Port=2
  Dot Product1212 : Sum  OutDataTypeStr=single  SampleTime=6.02409638554217e-09
  Dot Product1212_pd1 : Delay  DelayLength=6
  Out1 : Outport
  wires:
  In1/1 -> Dot Product1212/1
  In2/1 -> Dot Product1212/2
  Dot Product1212/1 -> Dot Product1212_pd1/1
  Dot Product1212_pd1/1 -> Out1/1

== system gm_MATE_HDLsolver_myFirstCircuit/ForFPGA/Dot Product1213 ==
  In1 : Inport
  In2 : Inport  Port=2
  Dot Product1213 : Sum  OutDataTypeStr=single  SampleTime=6.02409638554217e-09
  Dot Product1213_pd1 : Delay  DelayLength=6
  Out1 : Outport
  wires:
  In1/1 -> Dot Product1213/1
  In2/1 -> Dot Product1213/2
  Dot Product1213/1 -> Dot Product1213_pd1/1
  Dot Product1213_pd1/1 -> Out1/1

== system gm_MATE_HDLsolver_myFirstCircuit/ForFPGA/Dot Product1214 ==
  In1 : Inport
  In2 : Inport  Port=2
  Dot Product1214 : Sum  OutDataTypeStr=single  SampleTime=6.02409638554217e-09
  Dot Product1214_pd1 : Delay  DelayLength=6
  Out1 : Outport
  wires:
  In1/1 -> Dot Product1214/1
  In2/1 -> Dot Product1214/2
  Dot Product1214/1 -> Dot Product1214_pd1/1
  Dot Product1214_pd1/1 -> Out1/1

== system gm_MATE_HDLsolver_myFirstCircuit/ForFPGA/Dot Product1215 ==
  In1 : Inport
  In2 : Inport  Port=2
  Dot Product1215 : Sum  OutDataTypeStr=single  SampleTime=6.02409638554217e-09
  Dot Product1215_pd1 : Delay  DelayLength=6
  Out1 : Outport
  wires:
  In1/1 -> Dot Product1215/1
  In2/1 -> Dot Product1215/2
  Dot Product1215/1 -> Dot Product1215_pd1/1
  Dot Product1215_pd1/1 -> Out1/1

== system gm_MATE_HDLsolver_myFirstCircuit/ForFPGA/Dot Product122 ==
  In1 : Inport
  In2 : Inport  Port=2
  Dot Product122 : Sum  OutDataTypeStr=single  SampleTime=6.02409638554217e-09
  Dot Product122_pd1 : Delay  DelayLength=6
  Out1 : Outport
  wires:
  In1/1 -> Dot Product122/1
  In2/1 -> Dot Product122/2
  Dot Product122/1 -> Dot Product122_pd1/1
  Dot Product122_pd1/1 -> Out1/1

== system gm_MATE_HDLsolver_myFirstCircuit/ForFPGA/Dot Product123 ==
  In1 : Inport
  In2 : Inport  Port=2
  Dot Product123 : Sum  OutDataTypeStr=single  SampleTime=6.02409638554217e-09
  Dot Product123_pd1 : Delay  DelayLength=6
  Out1 : Outport
  wires:
  In1/1 -> Dot Product123/1
  In2/1 -> Dot Product123/2
  Dot Product123/1 -> Dot Product123_pd1/1
  Dot Product123_pd1/1 -> Out1/1

== system gm_MATE_HDLsolver_myFirstCircuit/ForFPGA/Dot Product124 ==
  In1 : Inport
  In2 : Inport  Port=2
  Dot Product124 : Sum  OutDataTypeStr=single  SampleTime=6.02409638554217e-09
  Dot Product124_pd1 : Delay  DelayLength=6
  Out1 : Outport
  wires:
  In1/1 -> Dot Product124/1
  In2/1 -> Dot Product124/2
  Dot Product124/1 -> Dot Product124_pd1/1
  Dot Product124_pd1/1 -> Out1/1

== system gm_MATE_HDLsolver_myFirstCircuit/ForFPGA/Dot Product125 ==
  In1 : Inport
  In2 : Inport  Port=2
  Dot Product125 : Sum  OutDataTypeStr=single  SampleTime=6.02409638554217e-09
  Dot Product125_pd1 : Delay  DelayLength=6
  Out1 : Outport
  wires:
  In1/1 -> Dot Product125/1
  In2/1 -> Dot Product125/2
  Dot Product125/1 -> Dot Product125_pd1/1
  Dot Product125_pd1/1 -> Out1/1

== system gm_MATE_HDLsolver_myFirstCircuit/ForFPGA/Dot Product126 ==
  In1 : Inport
  In2 : Inport  Port=2
  Dot Product126 : Sum  OutDataTypeStr=single  SampleTime=6.02409638554217e-09
  Dot Product126_pd1 : Delay  DelayLength=6
  Out1 : Outport
  wires:
  In1/1 -> Dot Product126/1
  In2/1 -> Dot Product126/2
  Dot Product126/1 -> Dot Product126_pd1/1
  Dot Product126_pd1/1 -> Out1/1

== system gm_MATE_HDLsolver_myFirstCircuit/ForFPGA/Dot Product127 ==
  In1 : Inport
  In2 : Inport  Port=2
  Dot Product127 : Sum  OutDataTypeStr=single  SampleTime=6.02409638554217e-09
  Dot Product127_pd1 : Delay  DelayLength=6
  Out1 : Outport
  wires:
  In1/1 -> Dot Product127/1
  In2/1 -> Dot Product127/2
  Dot Product127/1 -> Dot Product127_pd1/1
  Dot Product127_pd1/1 -> Out1/1

== system gm_MATE_HDLsolver_myFirstCircuit/ForFPGA/Dot Product128 ==
  In1 : Inport
  In2 : Inport  Port=2
  Dot Product128 : Sum  OutDataTypeStr=single  SampleTime=6.02409638554217e-09
  Dot Product128_pd1 : Delay  DelayLength=6
  Out1 : Outport
  wires:
  In1/1 -> Dot Product128/1
  In2/1 -> Dot Product128/2
  Dot Product128/1 -> Dot Product128_pd1/1
  Dot Product128_pd1/1 -> Out1/1

== system gm_MATE_HDLsolver_myFirstCircuit/ForFPGA/Dot Product129 ==
  In1 : Inport
  In2 : Inport  Port=2
  Dot Product129 : Sum  OutDataTypeStr=single  SampleTime=6.02409638554217e-09
  Dot Product129_pd1 : Delay  DelayLength=6
  Out1 : Outport
  wires:
  In1/1 -> Dot Product129/1
  In2/1 -> Dot Product129/2
  Dot Product129/1 -> Dot Product129_pd1/1
  Dot Product129_pd1/1 -> Out1/1

== system gm_MATE_HDLsolver_myFirstCircuit/ForFPGA/Dot Product13 ==
  In1 : Inport
  In2 : Inport  Port=2
  Dot Product13 : Sum  OutDataTypeStr=single  SampleTime=6.02409638554217e-09
  Dot Product13_pd1 : Delay  DelayLength=6
  Out1 : Outport
  wires:
  In1/1 -> Dot Product13/1
  In2/1 -> Dot Product13/2
  Dot Product13/1 -> Dot Product13_pd1/1
  Dot Product13_pd1/1 -> Out1/1

== system gm_MATE_HDLsolver_myFirstCircuit/ForFPGA/Dot Product131 ==
  In1 : Inport
  In2 : Inport  Port=2
  Dot Product131 : Sum  OutDataTypeStr=single  SampleTime=6.02409638554217e-09
  Dot Product131_pd1 : Delay  DelayLength=6
  Out1 : Outport
  wires:
  In1/1 -> Dot Product131/1
  In2/1 -> Dot Product131/2
  Dot Product131/1 -> Dot Product131_pd1/1
  Dot Product131_pd1/1 -> Out1/1

== system gm_MATE_HDLsolver_myFirstCircuit/ForFPGA/Dot Product1310 ==
  In1 : Inport
  In2 : Inport  Port=2
  Dot Product1310 : Sum  OutDataTypeStr=single  SampleTime=6.02409638554217e-09
  Dot Product1310_pd1 : Delay  DelayLength=6
  Out1 : Outport
  wires:
  In1/1 -> Dot Product1310/1
  In2/1 -> Dot Product1310/2
  Dot Product1310/1 -> Dot Product1310_pd1/1
  Dot Product1310_pd1/1 -> Out1/1

== system gm_MATE_HDLsolver_myFirstCircuit/ForFPGA/Dot Product1311 ==
  In1 : Inport
  In2 : Inport  Port=2
  Dot Product1311 : Sum  OutDataTypeStr=single  SampleTime=6.02409638554217e-09
  Dot Product1311_pd1 : Delay  DelayLength=6
  Out1 : Outport
  wires:
  In1/1 -> Dot Product1311/1
  In2/1 -> Dot Product1311/2
  Dot Product1311/1 -> Dot Product1311_pd1/1
  Dot Product1311_pd1/1 -> Out1/1

== system gm_MATE_HDLsolver_myFirstCircuit/ForFPGA/Dot Product1312 ==
  In1 : Inport
  In2 : Inport  Port=2
  Dot Product1312 : Sum  OutDataTypeStr=single  SampleTime=6.02409638554217e-09
  Dot Product1312_pd1 : Delay  DelayLength=6
  Out1 : Outport
  wires:
  In1/1 -> Dot Product1312/1
  In2/1 -> Dot Product1312/2
  Dot Product1312/1 -> Dot Product1312_pd1/1
  Dot Product1312_pd1/1 -> Out1/1

== system gm_MATE_HDLsolver_myFirstCircuit/ForFPGA/Dot Product1313 ==
  In1 : Inport
  In2 : Inport  Port=2
  Dot Product1313 : Sum  OutDataTypeStr=single  SampleTime=6.02409638554217e-09
  Dot Product1313_pd1 : Delay  DelayLength=6
  Out1 : Outport
  wires:
  In1/1 -> Dot Product1313/1
  In2/1 -> Dot Product1313/2
  Dot Product1313/1 -> Dot Product1313_pd1/1
  Dot Product1313_pd1/1 -> Out1/1

== system gm_MATE_HDLsolver_myFirstCircuit/ForFPGA/Dot Product1314 ==
  In1 : Inport
  In2 : Inport  Port=2
  Dot Product1314 : Sum  OutDataTypeStr=single  SampleTime=6.02409638554217e-09
  Dot Product1314_pd1 : Delay  DelayLength=6
  Out1 : Outport
  wires:
  In1/1 -> Dot Product1314/1
  In2/1 -> Dot Product1314/2
  Dot Product1314/1 -> Dot Product1314_pd1/1
  Dot Product1314_pd1/1 -> Out1/1

== system gm_MATE_HDLsolver_myFirstCircuit/ForFPGA/Dot Product1315 ==
  In1 : Inport
  In2 : Inport  Port=2
  Dot Product1315 : Sum  OutDataTypeStr=single  SampleTime=6.02409638554217e-09
  Dot Product1315_pd1 : Delay  DelayLength=6
  Out1 : Outport
  wires:
  In1/1 -> Dot Product1315/1
  In2/1 -> Dot Product1315/2
  Dot Product1315/1 -> Dot Product1315_pd1/1
  Dot Product1315_pd1/1 -> Out1/1

== system gm_MATE_HDLsolver_myFirstCircuit/ForFPGA/Dot Product132 ==
  In1 : Inport
  In2 : Inport  Port=2
  Dot Product132 : Sum  OutDataTypeStr=single  SampleTime=6.02409638554217e-09
  Dot Product132_pd1 : Delay  DelayLength=6
  Out1 : Outport
  wires:
  In1/1 -> Dot Product132/1
  In2/1 -> Dot Product132/2
  Dot Product132/1 -> Dot Product132_pd1/1
  Dot Product132_pd1/1 -> Out1/1

== system gm_MATE_HDLsolver_myFirstCircuit/ForFPGA/Dot Product133 ==
  In1 : Inport
  In2 : Inport  Port=2
  Dot Product133 : Sum  OutDataTypeStr=single  SampleTime=6.02409638554217e-09
  Dot Product133_pd1 : Delay  DelayLength=6
  Out1 : Outport
  wires:
  In1/1 -> Dot Product133/1
  In2/1 -> Dot Product133/2
  Dot Product133/1 -> Dot Product133_pd1/1
  Dot Product133_pd1/1 -> Out1/1

== system gm_MATE_HDLsolver_myFirstCircuit/ForFPGA/Dot Product134 ==
  In1 : Inport
  In2 : Inport  Port=2
  Dot Product134 : Sum  OutDataTypeStr=single  SampleTime=6.02409638554217e-09
  Dot Product134_pd1 : Delay  DelayLength=6
  Out1 : Outport
  wires:
  In1/1 -> Dot Product134/1
  In2/1 -> Dot Product134/2
  Dot Product134/1 -> Dot Product134_pd1/1
  Dot Product134_pd1/1 -> Out1/1

== system gm_MATE_HDLsolver_myFirstCircuit/ForFPGA/Dot Product135 ==
  In1 : Inport
  In2 : Inport  Port=2
  Dot Product135 : Sum  OutDataTypeStr=single  SampleTime=6.02409638554217e-09
  Dot Product135_pd1 : Delay  DelayLength=6
  Out1 : Outport
  wires:
  In1/1 -> Dot Product135/1
  In2/1 -> Dot Product135/2
  Dot Product135/1 -> Dot Product135_pd1/1
  Dot Product135_pd1/1 -> Out1/1

== system gm_MATE_HDLsolver_myFirstCircuit/ForFPGA/Dot Product136 ==
  In1 : Inport
  In2 : Inport  Port=2
  Dot Product136 : Sum  OutDataTypeStr=single  SampleTime=6.02409638554217e-09
  Dot Product136_pd1 : Delay  DelayLength=6
  Out1 : Outport
  wires:
  In1/1 -> Dot Product136/1
  In2/1 -> Dot Product136/2
  Dot Product136/1 -> Dot Product136_pd1/1
  Dot Product136_pd1/1 -> Out1/1

== system gm_MATE_HDLsolver_myFirstCircuit/ForFPGA/Dot Product137 ==
  In1 : Inport
  In2 : Inport  Port=2
  Dot Product137 : Sum  OutDataTypeStr=single  SampleTime=6.02409638554217e-09
  Dot Product137_pd1 : Delay  DelayLength=6
  Out1 : Outport
  wires:
  In1/1 -> Dot Product137/1
  In2/1 -> Dot Product137/2
  Dot Product137/1 -> Dot Product137_pd1/1
  Dot Product137_pd1/1 -> Out1/1

== system gm_MATE_HDLsolver_myFirstCircuit/ForFPGA/Dot Product138 ==
  In1 : Inport
  In2 : Inport  Port=2
  Dot Product138 : Sum  OutDataTypeStr=single  SampleTime=6.02409638554217e-09
  Dot Product138_pd1 : Delay  DelayLength=6
  Out1 : Outport
  wires:
  In1/1 -> Dot Product138/1
  In2/1 -> Dot Product138/2
  Dot Product138/1 -> Dot Product138_pd1/1
  Dot Product138_pd1/1 -> Out1/1

== system gm_MATE_HDLsolver_myFirstCircuit/ForFPGA/Dot Product139 ==
  In1 : Inport
  In2 : Inport  Port=2
  Dot Product139 : Sum  OutDataTypeStr=single  SampleTime=6.02409638554217e-09
  Dot Product139_pd1 : Delay  DelayLength=6
  Out1 : Outport
  wires:
  In1/1 -> Dot Product139/1
  In2/1 -> Dot Product139/2
  Dot Product139/1 -> Dot Product139_pd1/1
  Dot Product139_pd1/1 -> Out1/1

== system gm_MATE_HDLsolver_myFirstCircuit/ForFPGA/Dot Product14 ==
  In1 : Inport
  In2 : Inport  Port=2
  Dot Product14 : Sum  OutDataTypeStr=single  SampleTime=6.02409638554217e-09
  Dot Product14_pd1 : Delay  DelayLength=6
  Out1 : Outport
  wires:
  In1/1 -> Dot Product14/1
  In2/1 -> Dot Product14/2
  Dot Product14/1 -> Dot Product14_pd1/1
  Dot Product14_pd1/1 -> Out1/1

== system gm_MATE_HDLsolver_myFirstCircuit/ForFPGA/Dot Product141 ==
  In1 : Inport
  In2 : Inport  Port=2
  Dot Product141 : Sum  OutDataTypeStr=single  SampleTime=6.02409638554217e-09
  Dot Product141_pd1 : Delay  DelayLength=6
  Out1 : Outport
  wires:
  In1/1 -> Dot Product141/1
  In2/1 -> Dot Product141/2
  Dot Product141/1 -> Dot Product141_pd1/1
  Dot Product141_pd1/1 -> Out1/1

== system gm_MATE_HDLsolver_myFirstCircuit/ForFPGA/Dot Product1410 ==
  In1 : Inport
  In2 : Inport  Port=2
  Dot Product1410 : Sum  OutDataTypeStr=single  SampleTime=6.02409638554217e-09
  Dot Product1410_pd1 : Delay  DelayLength=6
  Out1 : Outport
  wires:
  In1/1 -> Dot Product1410/1
  In2/1 -> Dot Product1410/2
  Dot Product1410/1 -> Dot Product1410_pd1/1
  Dot Product1410_pd1/1 -> Out1/1

== system gm_MATE_HDLsolver_myFirstCircuit/ForFPGA/Dot Product1411 ==
  In1 : Inport
  In2 : Inport  Port=2
  Dot Product1411 : Sum  OutDataTypeStr=single  SampleTime=6.02409638554217e-09
  Dot Product1411_pd1 : Delay  DelayLength=6
  Out1 : Outport
  wires:
  In1/1 -> Dot Product1411/1
  In2/1 -> Dot Product1411/2
  Dot Product1411/1 -> Dot Product1411_pd1/1
  Dot Product1411_pd1/1 -> Out1/1
